simulink model "actuators_switch_states_monitor_func"  (R2021a)
settings: Solver=VariableStepAuto  StartTime=0.0  StopTime=10.0  RelTol=1e-3
settings Model: Creator=Intuito_PC  LastModifiedBy=Intuito_PC

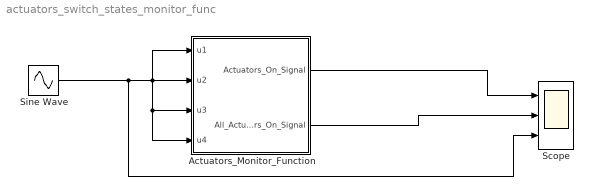
== system actuators_switch_states_monitor_func ==
  Actuators_Monitor_Function : MATLAB Function  TreatAsAtomicUnit=on
  Scope : Scope  NumInputPorts=3
  Sine Wave : Sin  SampleTime=0
  wires:
  Sine Wave/1 -> Scope/3, Actuators_Monitor_Function/4(u4), Actuators_Monitor_Function/3(u3), Actuators_Monitor_Function/1(u1), Actuators_Monitor_Function/2(u2)
  Actuators_Monitor_Function/1(Actuators_On_Signal) -> Scope/1
  Actuators_Monitor_Function/2(All_Actuators_On_Signal) -> Scope/2

== matlab function actuators_switch_states_monitor_func/Actuators_Monitor_Function ==
  data: u1 input; Actuators_On_Signal output; u2 input; u3 input; u4 input; All_Actuators_On_Signal output
function [Actuators_On_Signal, All_Actuators_On_Signal] = fcn(u1, u2, u3, u4)
% Initiate defaults
Actuators_On_Signal = 0;
All_Actuators_On_Signal = 0;
% Check actuators switch states
if (u1 + u2 + u3 + u4) < 1 
%     All_Actuators_On_Signal = 0; % Check if all actuators are on
    Actuators_On_Signal = 0; 
elseif (u1 + u2 + u3 + u4) > 0 && (u1 + u2 + u3 + u4) <= 3.1 
    Actuators_On_Signal = 1; % Check if an actuator is on
end
    if (u1 + u2 + u3 + u4) > 3.5
    All_Actuators_On_Signal = 1; % Check if all actuators are on
    else
       All_Actuators_On_Signal = 0; % Check if all actuators are on
end
end
